simulink model "ACCWithSensorFusionMdlRef"  (R2022b)
settings: Solver=FixedStepAuto  StartTime=0.0  StopTime=34  FixedStep=0.1  RelTol=1e-3
values from neighbouring files (symbols this model uses):
  default_spacing = 5    [helperACCSetUp.m]
  max_ac = 2    [helperACCSetUp.m]
  min_ac = -3    [helperACCSetUp.m]
  posSelector = [1,0,0,0,0,0; 0,0,1,0,0,0]    [helperACCSetUp.m]
  time_gap = 1.5    [helperACCSetUp.m]
  Ts = 0.1    [helperACCSetUp.m]
  v_set = 21.5    [helperACCSetUp.m]
  verr_gain = 0.5    [helperACCSetUp.m]
  vx_gain = 0.4    [helperACCSetUp.m]
  xerr_gain = 0.2    [helperACCSetUp.m]
libraries: mpcadaslib x1, trackingutilitieslib x1, drivinglib x1
settings Model: Creator=The MathWorks, Inc.  LastModifiedBy=The MathWorks, Inc.
settings SolverCC: AlgebraicLoopSolver=TrustRegion  MinimalZcImpactIntegration=on
settings DataIOCC: SaveOutput=off  SignalLogging=off  SaveTime=off  ReturnWorkspaceOutputs=off
settings OptimizationCC: DefaultParameterBehavior=Inlined  InlineInvariantSignals=on  PassReuseOutputArgsAs=Individual arguments  ZeroExternalMemoryAtStartup=off  ZeroInternalMemoryAtStartup=off  OptimizeBlockOrder=speed  EfficientTunableParamExpr=on
settings DebuggingCC: ParameterTunabilityLossMsg=error  UnconnectedInputMsg=warning  UnconnectedOutputMsg=warning  UnconnectedLineMsg=warning  SFMachineParentedDataDiag=warning  ArithmeticOperatorsInVariantConditions=warning
settings HardwareCC: ProdLongLongMode=on
settings ModelReferenceCC: EnableRefExpFcnMdlSchedulingChecks=on  PropagateVarSize=Only when enabling
settings SFSimCC: SimUseLocalCustomCode=off  MATLABDynamicMemAlloc=off  CustomCodeUndefinedFunction=UseInterfaceOnly  SimTargetLang=C++
settings RTWCC: Description=Embedded Coder  SystemTargetFile=ert.tlc  TemplateMakefile=ert_default_tmf  GenerateReport=on  RTWUseLocalCustomCode=off  BuildConfiguration=Faster Runs  IncludeHyperlinkInReport=on  LaunchReport=on  TargetLang=C++  GenerateTraceInfo=on  GenerateTraceReport=on  GenerateTraceReportSl=on  GenerateTraceReportSf=on  GenerateTraceReportEml=on  GenerateCodeMetricsReport=on  DLArmComputeVersion=19.05
settings CodeAppCC: ForceParamTrailComments=on  IgnoreCustomStorageClasses=off  MaxIdLength=63  OperatorAnnotations=on  SimulinkDataObjDesc=on  SFDataObjDesc=on  CustomSymbolStrFcn=$N$M$F  InsertBlockDesc=on
settings ERTTargetCC: TargetLangStandard=C++03 (ISO)  GenerateSampleERTMain=on  CombineSignalStateStructs=on  SuppressErrorStatus=on  CodeInterfacePackaging=C++ class  InlinedParameterPlacement=NonHierarchical  RootIOFormat=Structure reference  RTWCAPISignals=on  ERTCustomFileTemplate=example_file_process.tlc

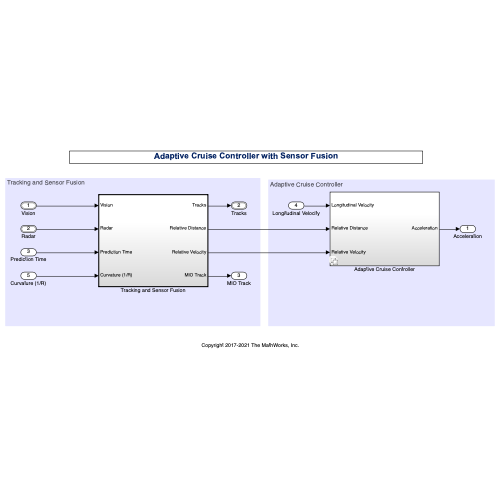
[thumbnail: Simulink's stored preview of the top-level diagram]
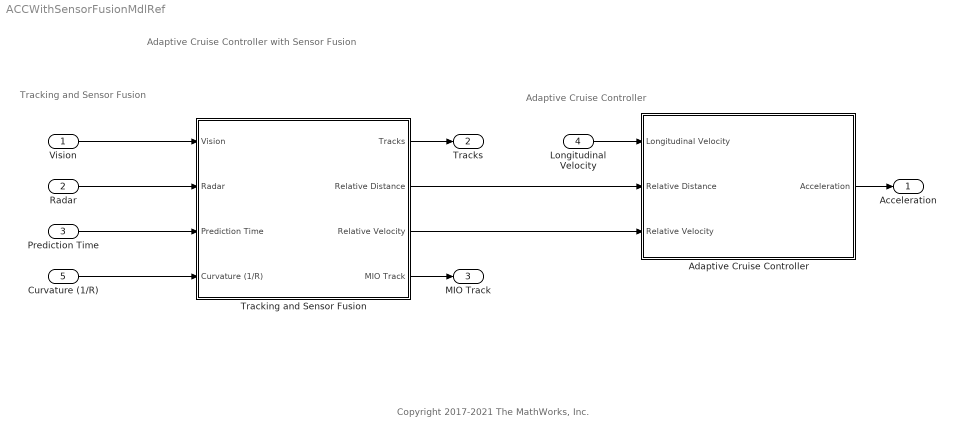
== system ACCWithSensorFusionMdlRef ==
  note: Adaptive Cruise Controller
  note: Tracking and Sensor Fusion
  note: Adaptive Cruise Controller with Sensor Fusion
  note: Copyright 2017-2021 The MathWorks, Inc.
  Vision : Inport  OutDataTypeStr=Bus: BusVision  PortDimensions=[1 1]  SampleTime=[0.10000000000000001,0]  BusOutputAsStruct=on
  Radar : Inport  Port=2  OutDataTypeStr=Bus: BusRadar  PortDimensions=[1 1]  SampleTime=[0.10000000000000001,0]  BusOutputAsStruct=on
  Prediction Time : Inport  Port=3  OutDataTypeStr=double  PortDimensions=[1 1]  SampleTime=[0.10000000000000001,0]  BusOutputAsStruct=on
  Longitudinal Velocity : Inport  Port=4  OutDataTypeStr=double  PortDimensions=1  SampleTime=[0.10000000000000001,0]
  Curvature (1/R) : Inport  Port=5  OutDataTypeStr=double  PortDimensions=[1 1]  SampleTime=[0.10000000000000001,0]  BusOutputAsStruct=on
  Adaptive Cruise Controller : Subsystem  Variant=on  VariantControl=Variant1
  Tracking and Sensor Fusion : Subsystem  TreatAsAtomicUnit=on
      settings: RTWFileNameOpts=Use function name
  "Acceleration " : Outport  OutDataTypeStr=double  PortDimensions=1  SampleTime=[0.10000000000000001,0]  VectorParamsAs1DForOutWhenUnconnected=off
  Tracks : Outport  Port=2  OutDataTypeStr=Bus:BusMultiObjectTracker1  PortDimensions=[1 1]  SampleTime=[0.10000000000000001,0]  VectorParamsAs1DForOutWhenUnconnected=off  BusOutputAsStruct=on
  MIO Track : Outport  Port=3  OutDataTypeStr=double  PortDimensions=1  SampleTime=[0.10000000000000001,0]  VectorParamsAs1DForOutWhenUnconnected=off  BusOutputAsStruct=on
  wires:
  Tracking and Sensor Fusion/1(Tracks) -> Tracks/1
  Vision/1 -> Tracking and Sensor Fusion/1(Vision)
  Radar/1 -> Tracking and Sensor Fusion/2(Radar)
  Prediction Time/1 -> Tracking and Sensor Fusion/3(Prediction Time)
  Curvature (1/R)/1 -> Tracking and Sensor Fusion/4(Curvature (1/R))
  Tracking and Sensor Fusion/4(MIO Track) -> MIO Track/1
  Longitudinal Velocity/1 -> Adaptive Cruise Controller/1("Longitudinal Velocity ")
  Tracking and Sensor Fusion/2(Relative Distance) -> Adaptive Cruise Controller/2(Relative Distance)
  Tracking and Sensor Fusion/3(Relative Velocity) -> Adaptive Cruise Controller/3("Relative Velocity ")
  Adaptive Cruise Controller/1(" Acceleration") -> "Acceleration "/1

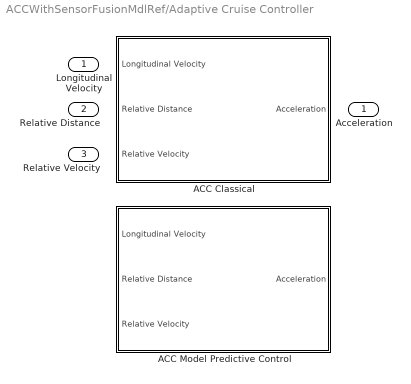
== system ACCWithSensorFusionMdlRef/Adaptive Cruise Controller ==
  "Longitudinal Velocity " : Inport
  Relative Distance : Inport  Port=2
  "Relative Velocity " : Inport  Port=3
  ACC Classical : Subsystem  TreatAsAtomicUnit=on  VariantControl=controller_type == 1
      settings: RTWFileNameOpts=Use function name
  ACC Model Predictive Control : Subsystem  TreatAsAtomicUnit=on  VariantControl=controller_type == 2
      settings: RTWFileNameOpts=Use function name
  " Acceleration" : Outport  VectorParamsAs1DForOutWhenUnconnected=off

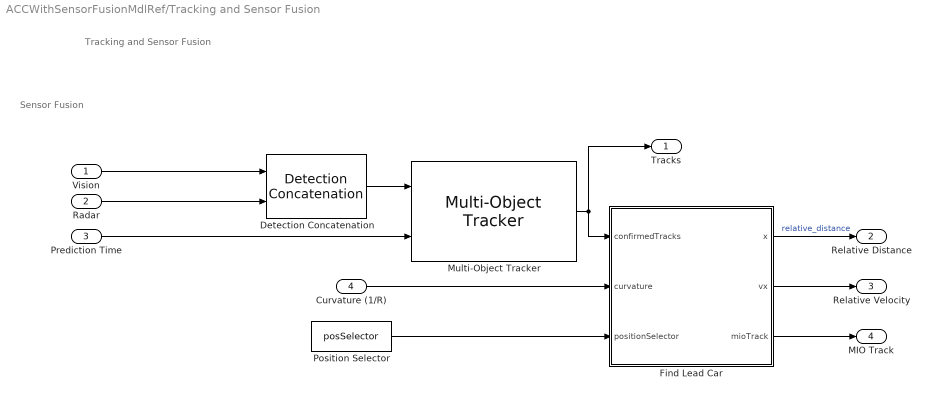
== system ACCWithSensorFusionMdlRef/Tracking and Sensor Fusion ==
  note: Sensor Fusion
  note: Tracking and Sensor Fusion
  Vision : Inport  OutDataTypeStr=Bus: BusVision  PortDimensions=[1 1]  SampleTime=[0.10000000000000001,0]  BusOutputAsStruct=on
  Radar : Inport  Port=2  OutDataTypeStr=Bus: BusRadar  PortDimensions=[1 1]  SampleTime=[0.10000000000000001,0]  BusOutputAsStruct=on
  Prediction Time : Inport  Port=3  OutDataTypeStr=double  PortDimensions=[1 1]  SampleTime=[0.10000000000000001,0]  BusOutputAsStruct=on
  Curvature (1/R) : Inport  Port=4  OutDataTypeStr=double  PortDimensions=[1 1]  SampleTime=[0.10000000000000001,0]  BusOutputAsStruct=on
  Detection Concatenation : trackingutilitieslib/Detection Concatenation  NumInputs=2  BusNameSource=Auto  BusName=BusDetectionConcatenation  SimulateUsing=Interpreted execution
  Find Lead Car : MATLAB Function  TreatAsAtomicUnit=on
  Multi-Object Tracker : drivinglib/Multi-Object Tracker  TrackerIndex=uint32( 0 )  FilterInitializationFcn=initcvekf  AssignmentThreshold=assigThresh  ConfirmationThreshold=[ 2, 3 ]  DeletionThreshold=[ 5, 5 ]  MaxNumTracks=numTracks  MaxNumSensors=numSensors  OOSMHandling=Terminate  StateParametersSimulink=struct  HasStateParametersInput=off  TimeInputSource=Input port  HasCostMatrixInput=off  HasDetectableTrackIDsInput=off  BusNameSource=Property  BusName=BusMultiObjectTracker1  TentativeTracksOutputPort=off  AllTracksOutputPort=off  SimulateUsing=Interpreted execution
  Position Selector : Constant  Value=posSelector
  Tracks : Outport  OutDataTypeStr=Bus:BusMultiObjectTracker1  PortDimensions=[1 1]  SampleTime=[0.10000000000000001,0]  VectorParamsAs1DForOutWhenUnconnected=off  BusOutputAsStruct=on
  Relative Distance : Outport  Port=2  VectorParamsAs1DForOutWhenUnconnected=off
  Relative Velocity : Outport  Port=3  VectorParamsAs1DForOutWhenUnconnected=off
  MIO Track : Outport  Port=4  VectorParamsAs1DForOutWhenUnconnected=off
  wires:
  Find Lead Car/3(mioTrack) -> MIO Track/1
  Radar/1 -> Detection Concatenation/2
  Vision/1 -> Detection Concatenation/1
  Prediction Time/1 -> Multi-Object Tracker/2
  Find Lead Car/2(vx) -> Relative Velocity/1
  Curvature (1/R)/1 -> Find Lead Car/2(curvature)
  Multi-Object Tracker/1 -> Find Lead Car/1(confirmedTracks), Tracks/1
  Detection Concatenation/1 -> Multi-Object Tracker/1
  Find Lead Car/1(x) -> Relative Distance/1  "relative_distance"
  Position Selector/1 -> Find Lead Car/3(positionSelector)

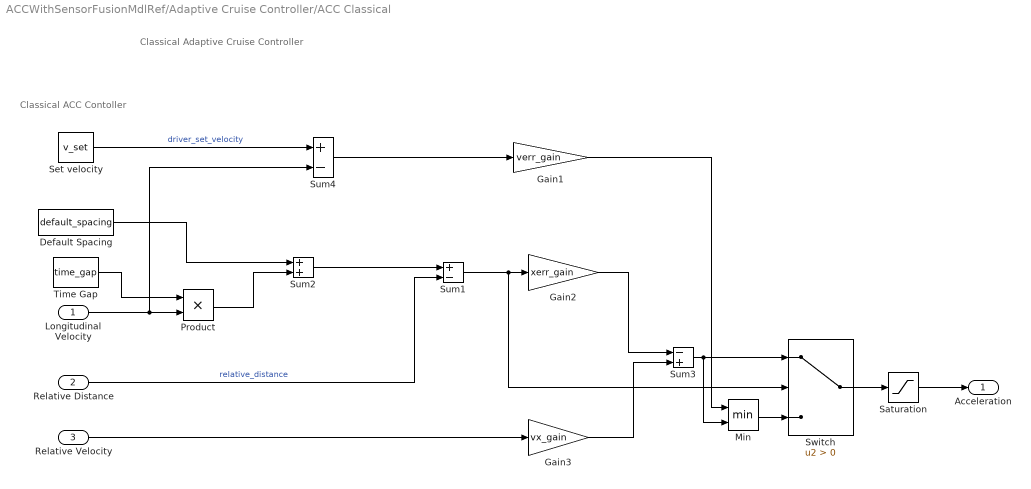
== system ACCWithSensorFusionMdlRef/Adaptive Cruise Controller/ACC Classical ==
  note: Classical ACC Contoller
  note: Classical Adaptive Cruise Controller
  Longitudinal Velocity : Inport
  Relative Distance : Inport  Port=2
  Relative Velocity : Inport  Port=3
  Default Spacing : Constant  Value=default_spacing  SampleTime=Ts
  Gain1 : Gain  Gain=verr_gain
  Gain2 : Gain  Gain=xerr_gain
  Gain3 : Gain  Gain=vx_gain
  Min : MinMax  Inputs=2
  Product : Product
  Saturation : Saturate  UpperLimit=max_ac  LowerLimit=min_ac
  Set velocity : Constant  Value=v_set  SampleTime=Ts
  Sum1 : Sum  Inputs=+-
  Sum2 : Sum
  Sum3 : Sum  Inputs=-+
  Sum4 : Sum  Inputs=+-
  Switch : Switch  Criteria=u2 > Threshold  SaturateOnIntegerOverflow=off  InputSameDT=off
  Time Gap : Constant  Value=time_gap  SampleTime=Ts
  Acceleration : Outport  VectorParamsAs1DForOutWhenUnconnected=off
  wires:
  Longitudinal Velocity/1 -> Product/2, Sum4/2
  Default Spacing/1 -> Sum2/1
  Gain2/1 -> Sum3/1
  Sum4/1 -> Gain1/1
  Min/1 -> Switch/3
  Gain3/1 -> Sum3/2
  Switch/1 -> Saturation/1
  Relative Velocity/1 -> Gain3/1
  Time Gap/1 -> Product/1
  Saturation/1 -> Acceleration/1
  Product/1 -> Sum2/2
  Set velocity/1 -> Sum4/1  "driver_set_velocity"
  Sum3/1 -> Min/2, Switch/1
  Sum1/1 -> Switch/2, Gain2/1
  Gain1/1 -> Min/1
  Relative Distance/1 -> Sum1/2  "relative_distance"
  Sum2/1 -> Sum1/1

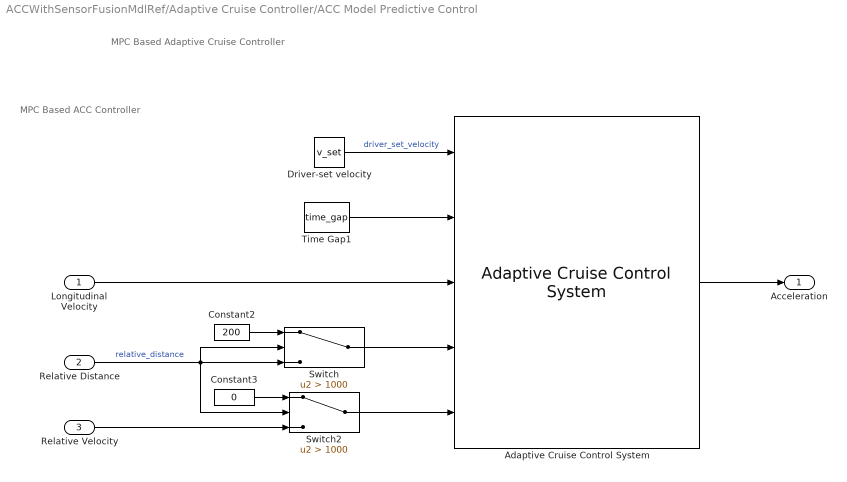
== system ACCWithSensorFusionMdlRef/Adaptive Cruise Controller/ACC Model Predictive Control ==
  note: MPC Based Adaptive Cruise Controller
  note: MPC Based ACC Controller
  Longitudinal Velocity : Inport
  Relative Distance : Inport  Port=2
  Relative Velocity : Inport  Port=3
  Adaptive Cruise Control System : mpcadaslib/Adaptive Cruise Control System  EgoModel=G  InitialEgoVelocity=v0_ego  DefaultSpacing=default_spacing  MaxVelocity=50  MinAcceleration=min_ac  amin_ext=off  MaxAcceleration=max_ac  amax_ext=off  Ts=Ts  PredictionHorizon=30  ControllerBehavior=0.5  suboptimal=off  maxiter=10  datatypeopt=double  optmode=off  trackmode=off
  Constant2 : Constant  Value=200  SampleTime=Ts
  Constant3 : Constant  Value=0  SampleTime=Ts
  Driver-set velocity : Constant  Value=v_set  SampleTime=Ts
  Switch : Switch  Criteria=u2 > Threshold  Threshold=1000  SaturateOnIntegerOverflow=off  InputSameDT=off
  Switch2 : Switch  Criteria=u2 > Threshold  Threshold=1000  SaturateOnIntegerOverflow=off  InputSameDT=off
  Time Gap1 : Constant  Value=time_gap  SampleTime=Ts
  Acceleration : Outport  OutDataTypeStr=double  PortDimensions=1  SampleTime=[0.10000000000000001,0]  VectorParamsAs1DForOutWhenUnconnected=off
  wires:
  Adaptive Cruise Control System/1 -> Acceleration/1
  Driver-set velocity/1 -> Adaptive Cruise Control System/1  "driver_set_velocity"
  Constant2/1 -> Switch/1
  Relative Distance/1 -> Switch/3, Switch2/2, Switch/2  "relative_distance"
  Constant3/1 -> Switch2/1
  Relative Velocity/1 -> Switch2/3
  Time Gap1/1 -> Adaptive Cruise Control System/2
  Longitudinal Velocity/1 -> Adaptive Cruise Control System/3
  Switch/1 -> Adaptive Cruise Control System/4
  Switch2/1 -> Adaptive Cruise Control System/5

== matlab function ACCWithSensorFusionMdlRef/Tracking and Sensor Fusion/Find Lead Car ==
  data: confirmedTracks input; x output double size=[1 1]; vx output size=[1 1]; curvature input; mioTrack output; positionSelector input
function [x,vx,mioTrack] = findLeadCar(confirmedTracks, curvature, positionSelector)
% This function finds the lead car: a car in front of the ego car that
% satisfies all the criteria below:
% * Within the ego car's lane.
% * In front of the ego car.
% * Closest to the ego car.

% Important notes:
% 1. If you change state definition, change the following:
%       State = [x;vx;y;vy;z;vz] (3D constant velocity)
numStates = 6;

% 2. The lane is defined using a parabolic model, where y=ax^2+bx+c. a is
%    equal to half the road curvature, b=0, and c is the offset of the lane
%    boundaries relative to the ego car. Overall lane width is assumed to
%    be 3.6m, typical highway lane width.
laneWidth = 3.6;

% 3. The ego car is assumed to be traveling in the middle of its lane, with
%    1.8m on each side of it. So, c=+1.8m for the left lane boundary and
%    -1.8m for the right lane boundary.
halfLaneWidth = laneWidth/2;

% Initialize outputs and parameters
maxX = cast(1000, 'like', confirmedTracks.Tracks(1).State);  % Far enough forward so that no track is expected to exceed this distance
trackID = 0;

for i = 1:confirmedTracks.NumTracks
    position = positionSelector * confirmedTracks.Tracks(i).State;
    x = position(1); % Longitudinal position of the track relative to ego
    y = position(2); % Lateral position of the track relative to ego
    
    if x < maxX && x > 0 % No point checking otherwise
        yleftLane  = polyval([curvature/2, 0,  halfLaneWidth],x); % Half a lane to the left
        yrightLane = polyval([curvature/2, 0, -halfLaneWidth],x); % Half a lane to the right
        
        % Find a new lead car
        if (yrightLane <= y) && (y <= yleftLane)
            maxX = x;
            trackID = i;
        end
    end
end

if trackID>0
    mioState = confirmedTracks.Tracks(trackID).State;
else
    mioState = inf(numStates,1,'like',confirmedTracks.Tracks(1).State);
end

% Output:
x = mioState(1);    % Longitudinal position of the lead car
vx = mioState(2);   % Longitudinal velocity of the lead car
mioTrack = trackID; % Index of the most important track
